simulink model "ParallelRC"  (R2012b)
settings: Solver=ode45  StartTime=0.0  StopTime=10.0  RelTol=1e-3
settings Model: Creator=sz609516  LastModifiedBy=sz609516
settings DataIOCC: SignalLoggingSaveFormat=ModelDataLogs
settings DebuggingCC: FcnCallInpInsideContextMsg=EnableAllAsWarning
settings GRTTargetCC: CombineOutputUpdateFcns=off  GRTInterface=on

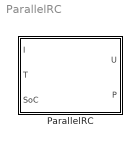
== system ParallelRC ==
  ParallelRC : Subsystem

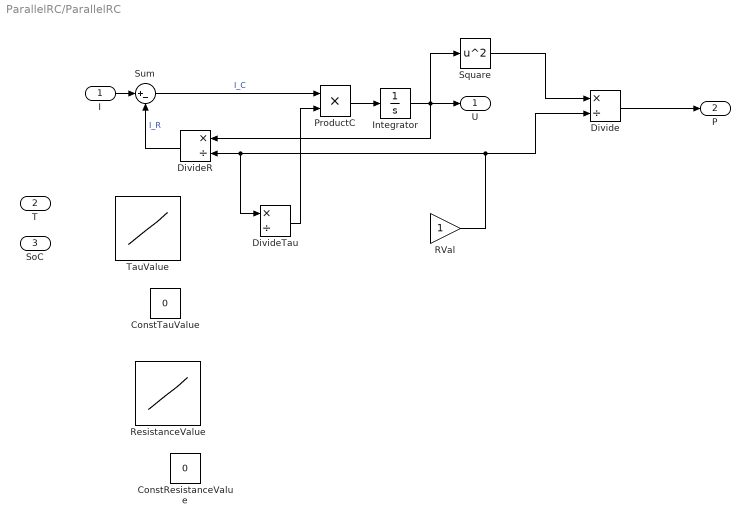
== system ParallelRC/ParallelRC ==
  I : Inport
  T : Inport  Port=2
  SoC : Inport  Port=3
  ConstResistanceValue : Constant  Value=0
  ConstTauValue : Constant  Value=0
  Divide : Product  Inputs=*/
  DivideR : Product  Inputs=*/
  DivideTau : Product  Inputs=*/
  Integrator : Integrator
  ProductC : Product  RndMeth=Zero
  RVal : Gain
  ResistanceValue : Lookup_n-D  Table=[1,2,3;4,5,6;7,8,9]  ExtrapMethod=Clip  RndMeth=Simplest  InputSameDT=on
  Square : Math  Operator=square  SaturateOnIntegerOverflow=on
  Sum : Sum  Inputs=|+-
  TauValue : Lookup_n-D  Table=[1,2,3;4,5,6;7,8,9]  ExtrapMethod=Clip  RndMeth=Simplest  InputSameDT=on
  U : Outport
  P : Outport  Port=2
  wires:
  I/1 -> Sum/1
  DivideR/1 -> Sum/2  "I_R"
  Sum/1 -> ProductC/1  "I_C"
  Square/1 -> Divide/1
  Divide/1 -> P/1
  ProductC/1 -> Integrator/1
  Integrator/1 -> Square/1, DivideR/1, U/1
  RVal/1 -> Divide/2, DivideR/2, DivideTau/1
  DivideTau/1 -> ProductC/2
